simulink model "a1be3ab"  (R2022a)
settings: Solver=VariableStepAuto  StartTime=0.0  StopTime=10  RelTol=1e-3
model workspace (MAT data in the model file):
  M_B = 5500
values from neighbouring files (symbols this model uses):
  b = 0.36    [a1be3ab.mat]
  c1 = 0.86    [a1be3ab.mat]
  c2 = 33.82    [a1be3ab.mat]
  c3 = 0.36    [a1be3ab.mat]
  g = 9.81    [a1be3ab.mat]
  J_R = 0.8    [a1be3ab.mat]
  m = 1500    [a1be3ab.mat]
  r_R = 0.3    [a1be3ab.mat]
libraries: simulink x1
settings Model: Creator=attit  LastModifiedBy=attit

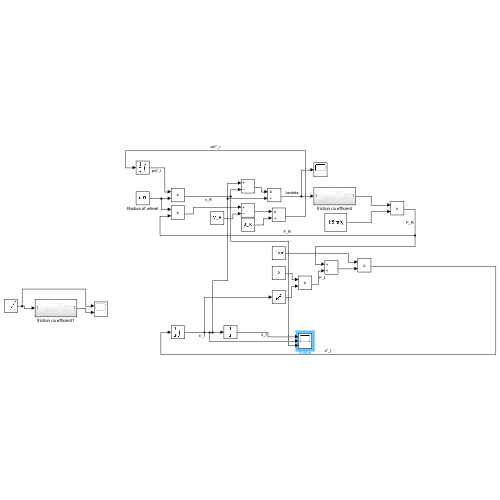
[thumbnail: Simulink's stored preview of the top-level diagram]
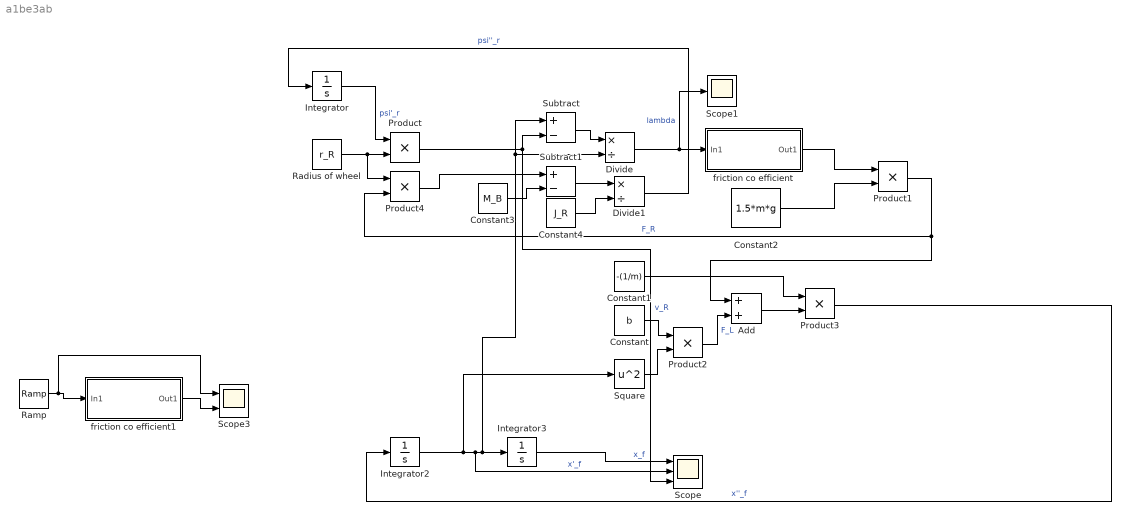
== system a1be3ab ==
  Add : Sum
  Constant : Constant  Value=b
  Constant1 : Constant  Value=-(1/m)
  Constant2 : Constant  Value=1.5*m*g
  Constant3 : Constant  Value=M_B
  Constant4 : Constant  Value=J_R
  Divide : Product  Inputs=*/
  Divide1 : Product  Inputs=*/
  Integrator : Integrator  InitialCondition=100  LimitOutput=on  LowerSaturationLimit=0
  Integrator2 : Integrator  InitialCondition=30  LimitOutput=on  LowerSaturationLimit=0
  Integrator3 : Integrator
  Product{,1..4} (5 alike) : Product
  Radius of wheel : Constant  Value=r_R
  Ramp : simulink/Sources/Ramp  slope=1  start=0  InitialOutput=0
  Scope : Scope  NumInputPorts=3
  Scope1 : Scope
  Scope3 : Scope  NumInputPorts=2
  Square : Math  Operator=square
  Subtract : Sum  Inputs=+-
  Subtract1 : Sum  Inputs=+-
  friction co efficient : Subsystem
  friction co efficient1 : Subsystem
  wires:
  Integrator/1 -> Product/1  "psi'_r"
  Divide1/1 -> Integrator/1  "psi''_r"
  Product3/1 -> Integrator2/1  "x''_f"
  Integrator2/1 -> Square/1, Scope/2, Divide/2, Subtract/1, Integrator3/1  "x'_f"
  Integrator3/1 -> Scope/1  "x_f"
  Radius of wheel/1 -> Product4/1, Product/2
  Product/1 -> Scope/3, Subtract/2  "v_R"
  Subtract/1 -> Divide/1
  Divide/1 -> Scope1/1, friction co efficient/1(In1)  "lambda"
  friction co efficient/1(Out1) -> Product1/1
  Constant2/1 -> Product1/2
  Square/1 -> Product2/2
  Constant/1 -> Product2/1
  Product1/1 -> Add/1, Product4/2  "F_R"
  Product2/1 -> Add/2  "F_L"
  Add/1 -> Product3/2
  Constant1/1 -> Product3/1
  Product4/1 -> Subtract1/1
  Constant3/1 -> Subtract1/2
  Subtract1/1 -> Divide1/1
  Constant4/1 -> Divide1/2
  Ramp/1 -> Scope3/1, friction co efficient1/1(In1)
  friction co efficient1/1(Out1) -> Scope3/2

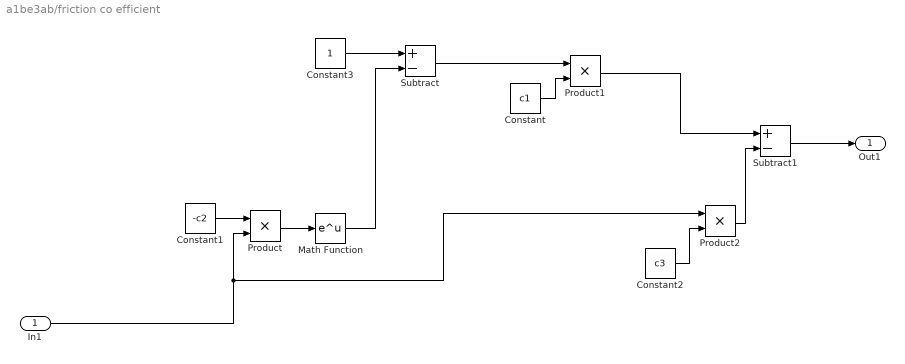
== system a1be3ab/friction co efficient ==
  In1 : Inport
  Constant : Constant  Value=c1
  Constant1 : Constant  Value=-c2
  Constant2 : Constant  Value=c3
  Constant3 : Constant
  Math Function : Math  SignedPower=on  RndMeth=Zero
  Product : Product
  Product1 : Product
  Product2 : Product
  Subtract : Sum  Inputs=+-
  Subtract1 : Sum  Inputs=+-
  Out1 : Outport
  wires:
  Constant1/1 -> Product/1
  In1/1 -> Product/2, Product2/1
  Product/1 -> Math Function/1
  Math Function/1 -> Subtract/2
  Constant3/1 -> Subtract/1
  Subtract/1 -> Product1/1
  Constant/1 -> Product1/2
  Constant2/1 -> Product2/2
  Product1/1 -> Subtract1/1
  Product2/1 -> Subtract1/2
  Subtract1/1 -> Out1/1

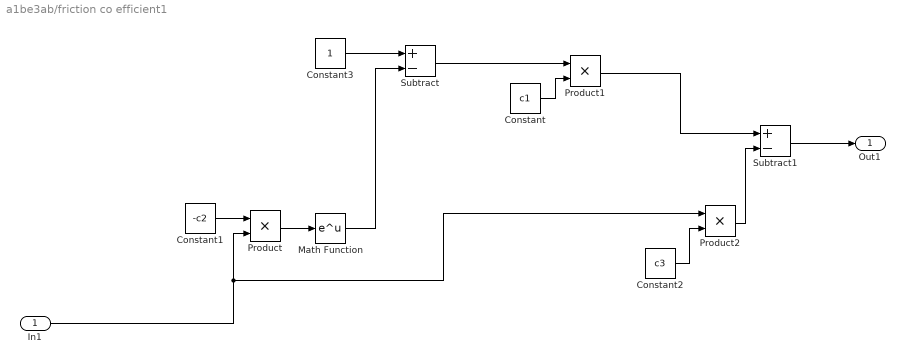
== system a1be3ab/friction co efficient1 ==
  In1 : Inport
  Constant : Constant  Value=c1
  Constant1 : Constant  Value=-c2
  Constant2 : Constant  Value=c3
  Constant3 : Constant
  Math Function : Math  SignedPower=on  RndMeth=Zero
  Product : Product
  Product1 : Product
  Product2 : Product
  Subtract : Sum  Inputs=+-
  Subtract1 : Sum  Inputs=+-
  Out1 : Outport
  wires:
  Subtract1/1 -> Out1/1
  Product2/1 -> Subtract1/2
  Product1/1 -> Subtract1/1
  Constant2/1 -> Product2/2
  Constant/1 -> Product1/2
  Subtract/1 -> Product1/1
  Constant3/1 -> Subtract/1
  Math Function/1 -> Subtract/2
  Product/1 -> Math Function/1
  In1/1 -> Product2/1, Product/2
  Constant1/1 -> Product/1
